simulink model "ACC_ISO_test_005_cs"  (Simulink 7.6)
settings: Solver=ode5  SolverMode=SingleTasking  StartTime=0.0  StopTime=inf  FixedStep=1/100  RelTol=1e-3
PreLoadFcn:
  | check_NUTS_defined;
  | 
  | assignin('base',['model_closed_' bdroot],false);addpath('../includes_ACC');
InitFcn:
  | PreScanExperimentInitFcn(bdroot)
StopFcn:
  | PreScanExperimentStopFcn(bdroot)
undefined symbols (not defined in the file): DiscIntNeverNeededParam, x_ini_VRML, y_ini_VRML, z_ini_VRML
libraries: simulink x25, PreScanSimulinkLibrary x12, simulink_extras x8, PreScanUsefulBlocks x5, simulink_need_slupdate x1
(part 2 of 7)

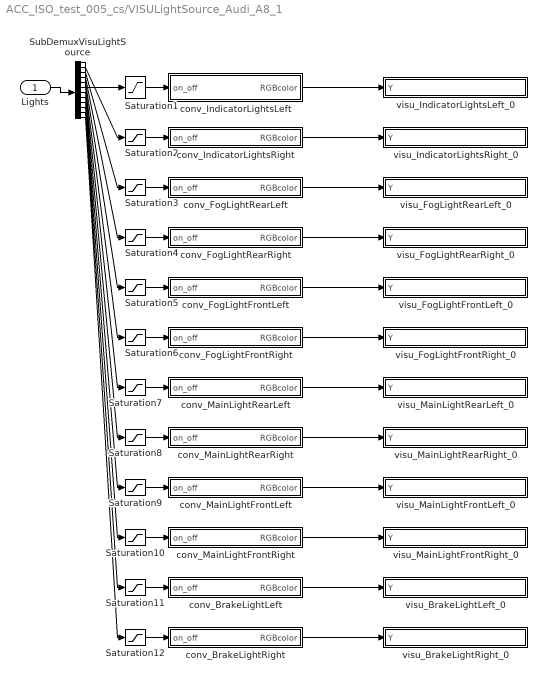
== system ACC_ISO_test_005_cs/VISULightSource_Audi_A8_1 ==
  Lights : Inport
  Saturation{1..12} (12 alike) : Saturate  UpperLimit=1  LowerLimit=0
  SubDemuxVisuLightSource : Demux  Outputs=12
  conv_BrakeLightLeft : Subsystem
  conv_BrakeLightRight : Subsystem
  conv_FogLightFrontLeft : Subsystem
  conv_FogLightFrontRight : Subsystem
  conv_FogLightRearLeft : Subsystem
  conv_FogLightRearRight : Subsystem
  conv_IndicatorLightsLeft : Subsystem
  conv_IndicatorLightsRight : Subsystem
  conv_MainLightFrontLeft : Subsystem
  conv_MainLightFrontRight : Subsystem
  conv_MainLightRearLeft : Subsystem
  conv_MainLightRearRight : Subsystem
  visu_BrakeLightLeft_0 : Subsystem  mask(ToSensorWorld){PortName=visu_BrakeLightLeft_0, PortIndex=203, PortWidth=16, TimeStep=1/100}
      mask prompts: PortName "Port Name [-]"; PortIndex "Index [-]"; PortWidth "Port Dimensions [-]"; TimeStep "Upload Period [s]"
      mask help: Sends signal(s) from Simulink to the Sensor World
      mask Help:
      | Sends signal(s) from Simulink to the Sensor World.
      | 
      | - Port Name [-]: specifies the name of the output terminal of the Simulink block.
      | - Index [-]: specifies the start position in the output vector sent to the Sensor World
      | - Port dimensions [-]: specifies the width (number of scalars) of the output port
      | - Upload period [s]: specifies the upload period (in seconds) of the port.
      mask Display: port_label('input', 1, PortName)
  visu_BrakeLightRight_0 : Subsystem  mask(ToSensorWorld){PortName=visu_BrakeLightRight_0, PortIndex=219, PortWidth=16, TimeStep=1/100}
      mask prompts: PortName "Port Name [-]"; PortIndex "Index [-]"; PortWidth "Port Dimensions [-]"; TimeStep "Upload Period [s]"
      mask help: Sends signal(s) from Simulink to the Sensor World
      mask Help:
      | Sends signal(s) from Simulink to the Sensor World.
      | 
      | - Port Name [-]: specifies the name of the output terminal of the Simulink block.
      | - Index [-]: specifies the start position in the output vector sent to the Sensor World
      | - Port dimensions [-]: specifies the width (number of scalars) of the output port
      | - Upload period [s]: specifies the upload period (in seconds) of the port.
      mask Display: port_label('input', 1, PortName)
  visu_FogLightFrontLeft_0 : Subsystem  mask(ToSensorWorld){PortName=visu_FogLightFrontLeft_0, PortIndex=107, PortWidth=16, TimeStep=1/100}
      mask prompts: PortName "Port Name [-]"; PortIndex "Index [-]"; PortWidth "Port Dimensions [-]"; TimeStep "Upload Period [s]"
      mask help: Sends signal(s) from Simulink to the Sensor World
      mask Help:
      | Sends signal(s) from Simulink to the Sensor World.
      | 
      | - Port Name [-]: specifies the name of the output terminal of the Simulink block.
      | - Index [-]: specifies the start position in the output vector sent to the Sensor World
      | - Port dimensions [-]: specifies the width (number of scalars) of the output port
      | - Upload period [s]: specifies the upload period (in seconds) of the port.
      mask Display: port_label('input', 1, PortName)
  visu_FogLightFrontRight_0 : Subsystem  mask(ToSensorWorld){PortName=visu_FogLightFrontRight_0, PortIndex=123, PortWidth=16, TimeStep=1/100}
      mask prompts: PortName "Port Name [-]"; PortIndex "Index [-]"; PortWidth "Port Dimensions [-]"; TimeStep "Upload Period [s]"
      mask help: Sends signal(s) from Simulink to the Sensor World
      mask Help:
      | Sends signal(s) from Simulink to the Sensor World.
      | 
      | - Port Name [-]: specifies the name of the output terminal of the Simulink block.
      | - Index [-]: specifies the start position in the output vector sent to the Sensor World
      | - Port dimensions [-]: specifies the width (number of scalars) of the output port
      | - Upload period [s]: specifies the upload period (in seconds) of the port.
      mask Display: port_label('input', 1, PortName)
  visu_FogLightRearLeft_0 : Subsystem  mask(ToSensorWorld){PortName=visu_FogLightRearLeft_0, PortIndex=75, PortWidth=16, TimeStep=1/100}
      mask prompts: PortName "Port Name [-]"; PortIndex "Index [-]"; PortWidth "Port Dimensions [-]"; TimeStep "Upload Period [s]"
      mask help: Sends signal(s) from Simulink to the Sensor World
      mask Help:
      | Sends signal(s) from Simulink to the Sensor World.
      | 
      | - Port Name [-]: specifies the name of the output terminal of the Simulink block.
      | - Index [-]: specifies the start position in the output vector sent to the Sensor World
      | - Port dimensions [-]: specifies the width (number of scalars) of the output port
      | - Upload period [s]: specifies the upload period (in seconds) of the port.
      mask Display: port_label('input', 1, PortName)
  visu_FogLightRearRight_0 : Subsystem  mask(ToSensorWorld){PortName=visu_FogLightRearRight_0, PortIndex=91, PortWidth=16, TimeStep=1/100}
      mask prompts: PortName "Port Name [-]"; PortIndex "Index [-]"; PortWidth "Port Dimensions [-]"; TimeStep "Upload Period [s]"
      mask help: Sends signal(s) from Simulink to the Sensor World
      mask Help:
      | Sends signal(s) from Simulink to the Sensor World.
      | 
      | - Port Name [-]: specifies the name of the output terminal of the Simulink block.
      | - Index [-]: specifies the start position in the output vector sent to the Sensor World
      | - Port dimensions [-]: specifies the width (number of scalars) of the output port
      | - Upload period [s]: specifies the upload period (in seconds) of the port.
      mask Display: port_label('input', 1, PortName)
  visu_IndicatorLightsLeft_0 : Subsystem  mask(ToSensorWorld){PortName=visu_IndicatorLightsLeft_0, PortIndex=43, PortWidth=16, TimeStep=1/100}
      mask prompts: PortName "Port Name [-]"; PortIndex "Index [-]"; PortWidth "Port Dimensions [-]"; TimeStep "Upload Period [s]"
      mask help: Sends signal(s) from Simulink to the Sensor World
      mask Help:
      | Sends signal(s) from Simulink to the Sensor World.
      | 
      | - Port Name [-]: specifies the name of the output terminal of the Simulink block.
      | - Index [-]: specifies the start position in the output vector sent to the Sensor World
      | - Port dimensions [-]: specifies the width (number of scalars) of the output port
      | - Upload period [s]: specifies the upload period (in seconds) of the port.
      mask Display: port_label('input', 1, PortName)
  visu_IndicatorLightsRight_0 : Subsystem  mask(ToSensorWorld){PortName=visu_IndicatorLightsRight_0, PortIndex=59, PortWidth=16, TimeStep=1/100}
      mask prompts: PortName "Port Name [-]"; PortIndex "Index [-]"; PortWidth "Port Dimensions [-]"; TimeStep "Upload Period [s]"
      mask help: Sends signal(s) from Simulink to the Sensor World
      mask Help:
      | Sends signal(s) from Simulink to the Sensor World.
      | 
      | - Port Name [-]: specifies the name of the output terminal of the Simulink block.
      | - Index [-]: specifies the start position in the output vector sent to the Sensor World
      | - Port dimensions [-]: specifies the width (number of scalars) of the output port
      | - Upload period [s]: specifies the upload period (in seconds) of the port.
      mask Display: port_label('input', 1, PortName)
  visu_MainLightFrontLeft_0 : Subsystem  mask(ToSensorWorld){PortName=visu_MainLightFrontLeft_0, PortIndex=171, PortWidth=16, TimeStep=1/100}
      mask prompts: PortName "Port Name [-]"; PortIndex "Index [-]"; PortWidth "Port Dimensions [-]"; TimeStep "Upload Period [s]"
      mask help: Sends signal(s) from Simulink to the Sensor World
      mask Help:
      | Sends signal(s) from Simulink to the Sensor World.
      | 
      | - Port Name [-]: specifies the name of the output terminal of the Simulink block.
      | - Index [-]: specifies the start position in the output vector sent to the Sensor World
      | - Port dimensions [-]: specifies the width (number of scalars) of the output port
      | - Upload period [s]: specifies the upload period (in seconds) of the port.
      mask Display: port_label('input', 1, PortName)
  visu_MainLightFrontRight_0 : Subsystem  mask(ToSensorWorld){PortName=visu_MainLightFrontRight_0, PortIndex=187, PortWidth=16, TimeStep=1/100}
      mask prompts: PortName "Port Name [-]"; PortIndex "Index [-]"; PortWidth "Port Dimensions [-]"; TimeStep "Upload Period [s]"
      mask help: Sends signal(s) from Simulink to the Sensor World
      mask Help:
      | Sends signal(s) from Simulink to the Sensor World.
      | 
      | - Port Name [-]: specifies the name of the output terminal of the Simulink block.
      | - Index [-]: specifies the start position in the output vector sent to the Sensor World
      | - Port dimensions [-]: specifies the width (number of scalars) of the output port
      | - Upload period [s]: specifies the upload period (in seconds) of the port.
      mask Display: port_label('input', 1, PortName)
  visu_MainLightRearLeft_0 : Subsystem  mask(ToSensorWorld){PortName=visu_MainLightRearLeft_0, PortIndex=139, PortWidth=16, TimeStep=1/100}
      mask prompts: PortName "Port Name [-]"; PortIndex "Index [-]"; PortWidth "Port Dimensions [-]"; TimeStep "Upload Period [s]"
      mask help: Sends signal(s) from Simulink to the Sensor World
      mask Help:
      | Sends signal(s) from Simulink to the Sensor World.
      | 
      | - Port Name [-]: specifies the name of the output terminal of the Simulink block.
      | - Index [-]: specifies the start position in the output vector sent to the Sensor World
      | - Port dimensions [-]: specifies the width (number of scalars) of the output port
      | - Upload period [s]: specifies the upload period (in seconds) of the port.
      mask Display: port_label('input', 1, PortName)
  visu_MainLightRearRight_0 : Subsystem  mask(ToSensorWorld){PortName=visu_MainLightRearRight_0, PortIndex=155, PortWidth=16, TimeStep=1/100}
      mask prompts: PortName "Port Name [-]"; PortIndex "Index [-]"; PortWidth "Port Dimensions [-]"; TimeStep "Upload Period [s]"
      mask help: Sends signal(s) from Simulink to the Sensor World
      mask Help:
      | Sends signal(s) from Simulink to the Sensor World.
      | 
      | - Port Name [-]: specifies the name of the output terminal of the Simulink block.
      | - Index [-]: specifies the start position in the output vector sent to the Sensor World
      | - Port dimensions [-]: specifies the width (number of scalars) of the output port
      | - Upload period [s]: specifies the upload period (in seconds) of the port.
      mask Display: port_label('input', 1, PortName)
  wires:
  Lights/1 -> SubDemuxVisuLightSource/1
  SubDemuxVisuLightSource/1 -> Saturation1/1
  Saturation1/1 -> conv_IndicatorLightsLeft/1(on_off)
  conv_IndicatorLightsLeft/1(RGBcolor) -> visu_IndicatorLightsLeft_0/1(Y)
  SubDemuxVisuLightSource/2 -> Saturation2/1
  Saturation2/1 -> conv_IndicatorLightsRight/1(on_off)
  conv_IndicatorLightsRight/1(RGBcolor) -> visu_IndicatorLightsRight_0/1(Y)
  SubDemuxVisuLightSource/3 -> Saturation3/1
  Saturation3/1 -> conv_FogLightRearLeft/1(on_off)
  conv_FogLightRearLeft/1(RGBcolor) -> visu_FogLightRearLeft_0/1(Y)
  SubDemuxVisuLightSource/4 -> Saturation4/1
  Saturation4/1 -> conv_FogLightRearRight/1(on_off)
  conv_FogLightRearRight/1(RGBcolor) -> visu_FogLightRearRight_0/1(Y)
  SubDemuxVisuLightSource/5 -> Saturation5/1
  Saturation5/1 -> conv_FogLightFrontLeft/1(on_off)
  conv_FogLightFrontLeft/1(RGBcolor) -> visu_FogLightFrontLeft_0/1(Y)
  SubDemuxVisuLightSource/6 -> Saturation6/1
  Saturation6/1 -> conv_FogLightFrontRight/1(on_off)
  conv_FogLightFrontRight/1(RGBcolor) -> visu_FogLightFrontRight_0/1(Y)
  SubDemuxVisuLightSource/7 -> Saturation7/1
  Saturation7/1 -> conv_MainLightRearLeft/1(on_off)
  conv_MainLightRearLeft/1(RGBcolor) -> visu_MainLightRearLeft_0/1(Y)
  SubDemuxVisuLightSource/8 -> Saturation8/1
  Saturation8/1 -> conv_MainLightRearRight/1(on_off)
  conv_MainLightRearRight/1(RGBcolor) -> visu_MainLightRearRight_0/1(Y)
  SubDemuxVisuLightSource/9 -> Saturation9/1
  Saturation9/1 -> conv_MainLightFrontLeft/1(on_off)
  conv_MainLightFrontLeft/1(RGBcolor) -> visu_MainLightFrontLeft_0/1(Y)
  SubDemuxVisuLightSource/10 -> Saturation10/1
  Saturation10/1 -> conv_MainLightFrontRight/1(on_off)
  conv_MainLightFrontRight/1(RGBcolor) -> visu_MainLightFrontRight_0/1(Y)
  SubDemuxVisuLightSource/11 -> Saturation11/1
  Saturation11/1 -> conv_BrakeLightLeft/1(on_off)
  conv_BrakeLightLeft/1(RGBcolor) -> visu_BrakeLightLeft_0/1(Y)
  SubDemuxVisuLightSource/12 -> Saturation12/1
  Saturation12/1 -> conv_BrakeLightRight/1(on_off)
  conv_BrakeLightRight/1(RGBcolor) -> visu_BrakeLightRight_0/1(Y)

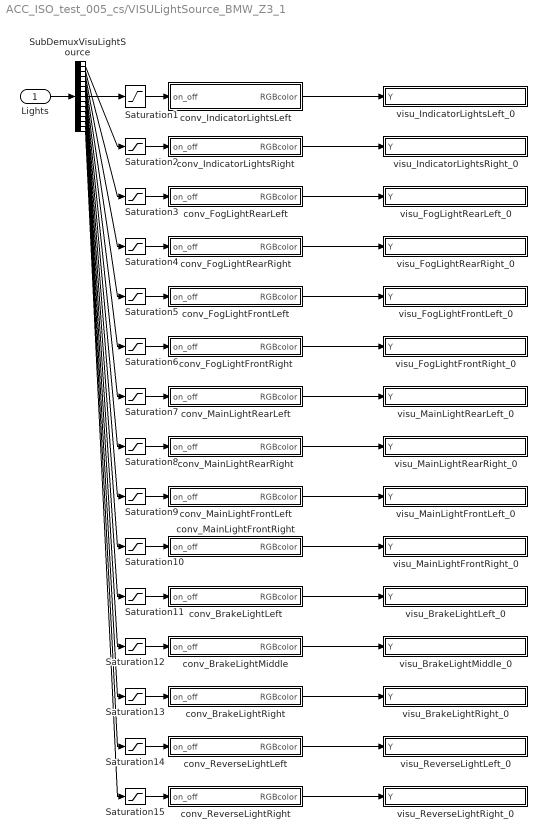
== system ACC_ISO_test_005_cs/VISULightSource_BMW_Z3_1 ==
  Lights : Inport
  Saturation{1..15} (15 alike) : Saturate  UpperLimit=1  LowerLimit=0
  SubDemuxVisuLightSource : Demux  Outputs=15
  conv_BrakeLightLeft : Subsystem
  conv_BrakeLightMiddle : Subsystem
  conv_BrakeLightRight : Subsystem
  conv_FogLightFrontLeft : Subsystem
  conv_FogLightFrontRight : Subsystem
  conv_FogLightRearLeft : Subsystem
  conv_FogLightRearRight : Subsystem
  conv_IndicatorLightsLeft : Subsystem
  conv_IndicatorLightsRight : Subsystem
  conv_MainLightFrontLeft : Subsystem
  conv_MainLightFrontRight : Subsystem
  conv_MainLightRearLeft : Subsystem
  conv_MainLightRearRight : Subsystem
  conv_ReverseLightLeft : Subsystem
  conv_ReverseLightRight : Subsystem
  visu_BrakeLightLeft_0 : Subsystem  mask(ToSensorWorld){PortName=visu_BrakeLightLeft_0, PortIndex=461, PortWidth=16, TimeStep=1/100}
      mask prompts: PortName "Port Name [-]"; PortIndex "Index [-]"; PortWidth "Port Dimensions [-]"; TimeStep "Upload Period [s]"
      mask help: Sends signal(s) from Simulink to the Sensor World
      mask Help:
      | Sends signal(s) from Simulink to the Sensor World.
      | 
      | - Port Name [-]: specifies the name of the output terminal of the Simulink block.
      | - Index [-]: specifies the start position in the output vector sent to the Sensor World
      | - Port dimensions [-]: specifies the width (number of scalars) of the output port
      | - Upload period [s]: specifies the upload period (in seconds) of the port.
      mask Display: port_label('input', 1, PortName)
  visu_BrakeLightMiddle_0 : Subsystem  mask(ToSensorWorld){PortName=visu_BrakeLightMiddle_0, PortIndex=477, PortWidth=16, TimeStep=1/100}
      mask prompts: PortName "Port Name [-]"; PortIndex "Index [-]"; PortWidth "Port Dimensions [-]"; TimeStep "Upload Period [s]"
      mask help: Sends signal(s) from Simulink to the Sensor World
      mask Help:
      | Sends signal(s) from Simulink to the Sensor World.
      | 
      | - Port Name [-]: specifies the name of the output terminal of the Simulink block.
      | - Index [-]: specifies the start position in the output vector sent to the Sensor World
      | - Port dimensions [-]: specifies the width (number of scalars) of the output port
      | - Upload period [s]: specifies the upload period (in seconds) of the port.
      mask Display: port_label('input', 1, PortName)
  visu_BrakeLightRight_0 : Subsystem  mask(ToSensorWorld){PortName=visu_BrakeLightRight_0, PortIndex=493, PortWidth=16, TimeStep=1/100}
      mask prompts: PortName "Port Name [-]"; PortIndex "Index [-]"; PortWidth "Port Dimensions [-]"; TimeStep "Upload Period [s]"
      mask help: Sends signal(s) from Simulink to the Sensor World
      mask Help:
      | Sends signal(s) from Simulink to the Sensor World.
      | 
      | - Port Name [-]: specifies the name of the output terminal of the Simulink block.
      | - Index [-]: specifies the start position in the output vector sent to the Sensor World
      | - Port dimensions [-]: specifies the width (number of scalars) of the output port
      | - Upload period [s]: specifies the upload period (in seconds) of the port.
      mask Display: port_label('input', 1, PortName)
  visu_FogLightFrontLeft_0 : Subsystem  mask(ToSensorWorld){PortName=visu_FogLightFrontLeft_0, PortIndex=365, PortWidth=16, TimeStep=1/100}
      mask prompts: PortName "Port Name [-]"; PortIndex "Index [-]"; PortWidth "Port Dimensions [-]"; TimeStep "Upload Period [s]"
      mask help: Sends signal(s) from Simulink to the Sensor World
      mask Help:
      | Sends signal(s) from Simulink to the Sensor World.
      | 
      | - Port Name [-]: specifies the name of the output terminal of the Simulink block.
      | - Index [-]: specifies the start position in the output vector sent to the Sensor World
      | - Port dimensions [-]: specifies the width (number of scalars) of the output port
      | - Upload period [s]: specifies the upload period (in seconds) of the port.
      mask Display: port_label('input', 1, PortName)
  visu_FogLightFrontRight_0 : Subsystem  mask(ToSensorWorld){PortName=visu_FogLightFrontRight_0, PortIndex=381, PortWidth=16, TimeStep=1/100}
      mask prompts: PortName "Port Name [-]"; PortIndex "Index [-]"; PortWidth "Port Dimensions [-]"; TimeStep "Upload Period [s]"
      mask help: Sends signal(s) from Simulink to the Sensor World
      mask Help:
      | Sends signal(s) from Simulink to the Sensor World.
      | 
      | - Port Name [-]: specifies the name of the output terminal of the Simulink block.
      | - Index [-]: specifies the start position in the output vector sent to the Sensor World
      | - Port dimensions [-]: specifies the width (number of scalars) of the output port
      | - Upload period [s]: specifies the upload period (in seconds) of the port.
      mask Display: port_label('input', 1, PortName)
  visu_FogLightRearLeft_0 : Subsystem  mask(ToSensorWorld){PortName=visu_FogLightRearLeft_0, PortIndex=333, PortWidth=16, TimeStep=1/100}
      mask prompts: PortName "Port Name [-]"; PortIndex "Index [-]"; PortWidth "Port Dimensions [-]"; TimeStep "Upload Period [s]"
      mask help: Sends signal(s) from Simulink to the Sensor World
      mask Help:
      | Sends signal(s) from Simulink to the Sensor World.
      | 
      | - Port Name [-]: specifies the name of the output terminal of the Simulink block.
      | - Index [-]: specifies the start position in the output vector sent to the Sensor World
      | - Port dimensions [-]: specifies the width (number of scalars) of the output port
      | - Upload period [s]: specifies the upload period (in seconds) of the port.
      mask Display: port_label('input', 1, PortName)
  visu_FogLightRearRight_0 : Subsystem  mask(ToSensorWorld){PortName=visu_FogLightRearRight_0, PortIndex=349, PortWidth=16, TimeStep=1/100}
      mask prompts: PortName "Port Name [-]"; PortIndex "Index [-]"; PortWidth "Port Dimensions [-]"; TimeStep "Upload Period [s]"
      mask help: Sends signal(s) from Simulink to the Sensor World
      mask Help:
      | Sends signal(s) from Simulink to the Sensor World.
      | 
      | - Port Name [-]: specifies the name of the output terminal of the Simulink block.
      | - Index [-]: specifies the start position in the output vector sent to the Sensor World
      | - Port dimensions [-]: specifies the width (number of scalars) of the output port
      | - Upload period [s]: specifies the upload period (in seconds) of the port.
      mask Display: port_label('input', 1, PortName)
  visu_IndicatorLightsLeft_0 : Subsystem  mask(ToSensorWorld){PortName=visu_IndicatorLightsLeft_0, PortIndex=301, PortWidth=16, TimeStep=1/100}
      mask prompts: PortName "Port Name [-]"; PortIndex "Index [-]"; PortWidth "Port Dimensions [-]"; TimeStep "Upload Period [s]"
      mask help: Sends signal(s) from Simulink to the Sensor World
      mask Help:
      | Sends signal(s) from Simulink to the Sensor World.
      | 
      | - Port Name [-]: specifies the name of the output terminal of the Simulink block.
      | - Index [-]: specifies the start position in the output vector sent to the Sensor World
      | - Port dimensions [-]: specifies the width (number of scalars) of the output port
      | - Upload period [s]: specifies the upload period (in seconds) of the port.
      mask Display: port_label('input', 1, PortName)
  visu_IndicatorLightsRight_0 : Subsystem  mask(ToSensorWorld){PortName=visu_IndicatorLightsRight_0, PortIndex=317, PortWidth=16, TimeStep=1/100}
      mask prompts: PortName "Port Name [-]"; PortIndex "Index [-]"; PortWidth "Port Dimensions [-]"; TimeStep "Upload Period [s]"
      mask help: Sends signal(s) from Simulink to the Sensor World
      mask Help:
      | Sends signal(s) from Simulink to the Sensor World.
      | 
      | - Port Name [-]: specifies the name of the output terminal of the Simulink block.
      | - Index [-]: specifies the start position in the output vector sent to the Sensor World
      | - Port dimensions [-]: specifies the width (number of scalars) of the output port
      | - Upload period [s]: specifies the upload period (in seconds) of the port.
      mask Display: port_label('input', 1, PortName)
  visu_MainLightFrontLeft_0 : Subsystem  mask(ToSensorWorld){PortName=visu_MainLightFrontLeft_0, PortIndex=429, PortWidth=16, TimeStep=1/100}
      mask prompts: PortName "Port Name [-]"; PortIndex "Index [-]"; PortWidth "Port Dimensions [-]"; TimeStep "Upload Period [s]"
      mask help: Sends signal(s) from Simulink to the Sensor World
      mask Help:
      | Sends signal(s) from Simulink to the Sensor World.
      | 
      | - Port Name [-]: specifies the name of the output terminal of the Simulink block.
      | - Index [-]: specifies the start position in the output vector sent to the Sensor World
      | - Port dimensions [-]: specifies the width (number of scalars) of the output port
      | - Upload period [s]: specifies the upload period (in seconds) of the port.
      mask Display: port_label('input', 1, PortName)
  visu_MainLightFrontRight_0 : Subsystem  mask(ToSensorWorld){PortName=visu_MainLightFrontRight_0, PortIndex=445, PortWidth=16, TimeStep=1/100}
      mask prompts: PortName "Port Name [-]"; PortIndex "Index [-]"; PortWidth "Port Dimensions [-]"; TimeStep "Upload Period [s]"
      mask help: Sends signal(s) from Simulink to the Sensor World
      mask Help:
      | Sends signal(s) from Simulink to the Sensor World.
      | 
      | - Port Name [-]: specifies the name of the output terminal of the Simulink block.
      | - Index [-]: specifies the start position in the output vector sent to the Sensor World
      | - Port dimensions [-]: specifies the width (number of scalars) of the output port
      | - Upload period [s]: specifies the upload period (in seconds) of the port.
      mask Display: port_label('input', 1, PortName)
  visu_MainLightRearLeft_0 : Subsystem  mask(ToSensorWorld){PortName=visu_MainLightRearLeft_0, PortIndex=397, PortWidth=16, TimeStep=1/100}
      mask prompts: PortName "Port Name [-]"; PortIndex "Index [-]"; PortWidth "Port Dimensions [-]"; TimeStep "Upload Period [s]"
      mask help: Sends signal(s) from Simulink to the Sensor World
      mask Help:
      | Sends signal(s) from Simulink to the Sensor World.
      | 
      | - Port Name [-]: specifies the name of the output terminal of the Simulink block.
      | - Index [-]: specifies the start position in the output vector sent to the Sensor World
      | - Port dimensions [-]: specifies the width (number of scalars) of the output port
      | - Upload period [s]: specifies the upload period (in seconds) of the port.
      mask Display: port_label('input', 1, PortName)
  visu_MainLightRearRight_0 : Subsystem  mask(ToSensorWorld){PortName=visu_MainLightRearRight_0, PortIndex=413, PortWidth=16, TimeStep=1/100}
      mask prompts: PortName "Port Name [-]"; PortIndex "Index [-]"; PortWidth "Port Dimensions [-]"; TimeStep "Upload Period [s]"
      mask help: Sends signal(s) from Simulink to the Sensor World
      mask Help:
      | Sends signal(s) from Simulink to the Sensor World.
      | 
      | - Port Name [-]: specifies the name of the output terminal of the Simulink block.
      | - Index [-]: specifies the start position in the output vector sent to the Sensor World
      | - Port dimensions [-]: specifies the width (number of scalars) of the output port
      | - Upload period [s]: specifies the upload period (in seconds) of the port.
      mask Display: port_label('input', 1, PortName)
  visu_ReverseLightLeft_0 : Subsystem  mask(ToSensorWorld){PortName=visu_ReverseLightLeft_0, PortIndex=509, PortWidth=16, TimeStep=1/100}
      mask prompts: PortName "Port Name [-]"; PortIndex "Index [-]"; PortWidth "Port Dimensions [-]"; TimeStep "Upload Period [s]"
      mask help: Sends signal(s) from Simulink to the Sensor World
      mask Help:
      | Sends signal(s) from Simulink to the Sensor World.
      | 
      | - Port Name [-]: specifies the name of the output terminal of the Simulink block.
      | - Index [-]: specifies the start position in the output vector sent to the Sensor World
      | - Port dimensions [-]: specifies the width (number of scalars) of the output port
      | - Upload period [s]: specifies the upload period (in seconds) of the port.
      mask Display: port_label('input', 1, PortName)
  visu_ReverseLightRight_0 : Subsystem  mask(ToSensorWorld){PortName=visu_ReverseLightRight_0, PortIndex=525, PortWidth=16, TimeStep=1/100}
      mask prompts: PortName "Port Name [-]"; PortIndex "Index [-]"; PortWidth "Port Dimensions [-]"; TimeStep "Upload Period [s]"
      mask help: Sends signal(s) from Simulink to the Sensor World
      mask Help:
      | Sends signal(s) from Simulink to the Sensor World.
      | 
      | - Port Name [-]: specifies the name of the output terminal of the Simulink block.
      | - Index [-]: specifies the start position in the output vector sent to the Sensor World
      | - Port dimensions [-]: specifies the width (number of scalars) of the output port
      | - Upload period [s]: specifies the upload period (in seconds) of the port.
      mask Display: port_label('input', 1, PortName)
  wires:
  Lights/1 -> SubDemuxVisuLightSource/1
  SubDemuxVisuLightSource/1 -> Saturation1/1
  Saturation1/1 -> conv_IndicatorLightsLeft/1(on_off)
  conv_IndicatorLightsLeft/1(RGBcolor) -> visu_IndicatorLightsLeft_0/1(Y)
  SubDemuxVisuLightSource/2 -> Saturation2/1
  Saturation2/1 -> conv_IndicatorLightsRight/1(on_off)
  conv_IndicatorLightsRight/1(RGBcolor) -> visu_IndicatorLightsRight_0/1(Y)
  SubDemuxVisuLightSource/3 -> Saturation3/1
  Saturation3/1 -> conv_FogLightRearLeft/1(on_off)
  conv_FogLightRearLeft/1(RGBcolor) -> visu_FogLightRearLeft_0/1(Y)
  SubDemuxVisuLightSource/4 -> Saturation4/1
  Saturation4/1 -> conv_FogLightRearRight/1(on_off)
  conv_FogLightRearRight/1(RGBcolor) -> visu_FogLightRearRight_0/1(Y)
  SubDemuxVisuLightSource/5 -> Saturation5/1
  Saturation5/1 -> conv_FogLightFrontLeft/1(on_off)
  conv_FogLightFrontLeft/1(RGBcolor) -> visu_FogLightFrontLeft_0/1(Y)
  SubDemuxVisuLightSource/6 -> Saturation6/1
  Saturation6/1 -> conv_FogLightFrontRight/1(on_off)
  conv_FogLightFrontRight/1(RGBcolor) -> visu_FogLightFrontRight_0/1(Y)
  SubDemuxVisuLightSource/7 -> Saturation7/1
  Saturation7/1 -> conv_MainLightRearLeft/1(on_off)
  conv_MainLightRearLeft/1(RGBcolor) -> visu_MainLightRearLeft_0/1(Y)
  SubDemuxVisuLightSource/8 -> Saturation8/1
  Saturation8/1 -> conv_MainLightRearRight/1(on_off)
  conv_MainLightRearRight/1(RGBcolor) -> visu_MainLightRearRight_0/1(Y)
  SubDemuxVisuLightSource/9 -> Saturation9/1
  Saturation9/1 -> conv_MainLightFrontLeft/1(on_off)
  conv_MainLightFrontLeft/1(RGBcolor) -> visu_MainLightFrontLeft_0/1(Y)
  SubDemuxVisuLightSource/10 -> Saturation10/1
  Saturation10/1 -> conv_MainLightFrontRight/1(on_off)
  conv_MainLightFrontRight/1(RGBcolor) -> visu_MainLightFrontRight_0/1(Y)
  SubDemuxVisuLightSource/11 -> Saturation11/1
  Saturation11/1 -> conv_BrakeLightLeft/1(on_off)
  conv_BrakeLightLeft/1(RGBcolor) -> visu_BrakeLightLeft_0/1(Y)
  SubDemuxVisuLightSource/12 -> Saturation12/1
  Saturation12/1 -> conv_BrakeLightMiddle/1(on_off)
  conv_BrakeLightMiddle/1(RGBcolor) -> visu_BrakeLightMiddle_0/1(Y)
  SubDemuxVisuLightSource/13 -> Saturation13/1
  Saturation13/1 -> conv_BrakeLightRight/1(on_off)
  conv_BrakeLightRight/1(RGBcolor) -> visu_BrakeLightRight_0/1(Y)
  SubDemuxVisuLightSource/14 -> Saturation14/1
  Saturation14/1 -> conv_ReverseLightLeft/1(on_off)
  conv_ReverseLightLeft/1(RGBcolor) -> visu_ReverseLightLeft_0/1(Y)
  SubDemuxVisuLightSource/15 -> Saturation15/1
  Saturation15/1 -> conv_ReverseLightRight/1(on_off)
  conv_ReverseLightRight/1(RGBcolor) -> visu_ReverseLightRight_0/1(Y)

== system ACC_ISO_test_005_cs/VISUSteer_Audi_A8_1 ==
  Steer : Inport
  Demux3 : Demux  Outputs=[1 1]
  Saturation : Saturate  UpperLimit=30  LowerLimit=-5
  Saturation1 : Saturate  UpperLimit=720  LowerLimit=-720
  conv_SteeringColumn : Subsystem
  conv_SteeringWheel : Subsystem
  visu_SteeringColumn : Subsystem  mask(ToSensorWorld){PortName=visu_SteeringColumn_0, PortIndex=239, PortWidth=4, TimeStep=1/100}
      mask prompts: PortName "Port Name [-]"; PortIndex "Index [-]"; PortWidth "Port Dimensions [-]"; TimeStep "Upload Period [s]"
      mask help: Sends signal(s) from Simulink to the Sensor World
      mask Help:
      | Sends signal(s) from Simulink to the Sensor World.
      | 
      | - Port Name [-]: specifies the name of the output terminal of the Simulink block.
      | - Index [-]: specifies the start position in the output vector sent to the Sensor World
      | - Port dimensions [-]: specifies the width (number of scalars) of the output port
      | - Upload period [s]: specifies the upload period (in seconds) of the port.
      mask Display: port_label('input', 1, PortName)
  visu_SteeringWheel : Subsystem  mask(ToSensorWorld){PortName=visu_SteeringWheel_0, PortIndex=235, PortWidth=4, TimeStep=1/100}
      mask prompts: PortName "Port Name [-]"; PortIndex "Index [-]"; PortWidth "Port Dimensions [-]"; TimeStep "Upload Period [s]"
      mask help: Sends signal(s) from Simulink to the Sensor World
      mask Help:
      | Sends signal(s) from Simulink to the Sensor World.
      | 
      | - Port Name [-]: specifies the name of the output terminal of the Simulink block.
      | - Index [-]: specifies the start position in the output vector sent to the Sensor World
      | - Port dimensions [-]: specifies the width (number of scalars) of the output port
      | - Upload period [s]: specifies the upload period (in seconds) of the port.
      mask Display: port_label('input', 1, PortName)
  wires:
  conv_SteeringColumn/1(QuaternionVisu [rad]) -> visu_SteeringColumn/1(Y)
  conv_SteeringWheel/1(QuaternionVisu [rad]) -> visu_SteeringWheel/1(Y)
  Demux3/2 -> Saturation/1
  Demux3/1 -> Saturation1/1
  Saturation1/1 -> conv_SteeringWheel/1(angle [deg])
  Saturation/1 -> conv_SteeringColumn/1(angle [deg])
  Steer/1 -> Demux3/1

== system ACC_ISO_test_005_cs/VISUSteer_BMW_Z3_1 ==
  Steer : Inport
  Demux3 : Demux  Outputs=[1 1]
  Saturation : Saturate  UpperLimit=30  LowerLimit=-5
  Saturation1 : Saturate  UpperLimit=720  LowerLimit=-720
  conv_SteeringColumn : Subsystem
  conv_SteeringWheel : Subsystem
  visu_SteeringColumn : Subsystem  mask(ToSensorWorld){PortName=visu_SteeringColumn_0, PortIndex=545, PortWidth=4, TimeStep=1/100}
      mask prompts: PortName "Port Name [-]"; PortIndex "Index [-]"; PortWidth "Port Dimensions [-]"; TimeStep "Upload Period [s]"
      mask help: Sends signal(s) from Simulink to the Sensor World
      mask Help:
      | Sends signal(s) from Simulink to the Sensor World.
      | 
      | - Port Name [-]: specifies the name of the output terminal of the Simulink block.
      | - Index [-]: specifies the start position in the output vector sent to the Sensor World
      | - Port dimensions [-]: specifies the width (number of scalars) of the output port
      | - Upload period [s]: specifies the upload period (in seconds) of the port.
      mask Display: port_label('input', 1, PortName)
  visu_SteeringWheel : Subsystem  mask(ToSensorWorld){PortName=visu_SteeringWheel_0, PortIndex=541, PortWidth=4, TimeStep=1/100}
      mask prompts: PortName "Port Name [-]"; PortIndex "Index [-]"; PortWidth "Port Dimensions [-]"; TimeStep "Upload Period [s]"
      mask help: Sends signal(s) from Simulink to the Sensor World
      mask Help:
      | Sends signal(s) from Simulink to the Sensor World.
      | 
      | - Port Name [-]: specifies the name of the output terminal of the Simulink block.
      | - Index [-]: specifies the start position in the output vector sent to the Sensor World
      | - Port dimensions [-]: specifies the width (number of scalars) of the output port
      | - Upload period [s]: specifies the upload period (in seconds) of the port.
      mask Display: port_label('input', 1, PortName)
  wires:
  conv_SteeringColumn/1(QuaternionVisu [rad]) -> visu_SteeringColumn/1(Y)
  conv_SteeringWheel/1(QuaternionVisu [rad]) -> visu_SteeringWheel/1(Y)
  Demux3/2 -> Saturation/1
  Demux3/1 -> Saturation1/1
  Saturation1/1 -> conv_SteeringWheel/1(angle [deg])
  Saturation/1 -> conv_SteeringColumn/1(angle [deg])
  Steer/1 -> Demux3/1

== system ACC_ISO_test_005_cs/VISUWheels_Audi_A8_1 ==
  Wheels : Inport
  Demux : Demux  Outputs=[3 3 3 3 3 3 3 3]
  Saturation{,2,4,6} (4 alike) : Saturate  UpperLimit=[0.2 0.2 0.5]  LowerLimit=[-0.2 -0.2 -0.5]
  Saturation{1,3,5,8} (4 alike) : Saturate  UpperLimit=[30 inf 30]  LowerLimit=[-30 -inf -30]
  conv_RotWheelFL : Subsystem
  conv_RotWheelFR : Subsystem
  conv_RotWheelRL : Subsystem
  conv_RotWheelRR : Subsystem
  conv_TransWheelFL : Subsystem  mask(Translation node configuration){tp=Front-Left Wheel, gains=off, Gain_xISO=1, Gain_yISO=1, Gain_zISO=1}
      mask prompts: tp "Type"; gains "Edit scaling factors?"; Gain_xISO "Scaling factor in x-direction (ISO-convention)"; Gain_yISO "Scaling factor in y-direction (ISO-convention)"; Gain_zISO "Scaling factor in z-direction (ISO-convention)"
      mask init:
      | Visu_ini_param('Audi_A8',tp);
      mask StyleString: popup(Front-Left Wheel|Front-Right Wheel|Rear-Left Wheel|Rear-Right Wheel|Left Seat|Right Seat),checkbox,edit,edit,edit
      mask CallbackString:
      | |if strcmp(get_param(gcb, 'gains'),'on')
      |     set_param(gcb,'MaskVisibilities',{'on','on','on','on','on'})
      | else
      |     set_param(gcb,'MaskVisibilities',{'on','on','off','off','off'})
      | end|||
  conv_TransWheelFR : Subsystem  mask(Translation node configuration){tp=Front-Right Wheel, gains=off, Gain_xISO=1, Gain_yISO=1, Gain_zISO=1}
      mask prompts: tp "Type"; gains "Edit scaling factors?"; Gain_xISO "Scaling factor in x-direction (ISO-convention)"; Gain_yISO "Scaling factor in y-direction (ISO-convention)"; Gain_zISO "Scaling factor in z-direction (ISO-convention)"
      mask init:
      | Visu_ini_param('Audi_A8',tp);
      mask StyleString: popup(Front-Left Wheel|Front-Right Wheel|Rear-Left Wheel|Rear-Right Wheel|Left Seat|Right Seat),checkbox,edit,edit,edit
      mask CallbackString:
      | |if strcmp(get_param(gcb, 'gains'),'on')
      |     set_param(gcb,'MaskVisibilities',{'on','on','on','on','on'})
      | else
      |     set_param(gcb,'MaskVisibilities',{'on','on','off','off','off'})
      | end|||
  conv_TransWheelRL : Subsystem  mask(Translation node configuration){tp=Rear-Left Wheel, gains=off, Gain_xISO=1, Gain_yISO=1, Gain_zISO=1}
      mask prompts: tp "Type"; gains "Edit scaling factors?"; Gain_xISO "Scaling factor in x-direction (ISO-convention)"; Gain_yISO "Scaling factor in y-direction (ISO-convention)"; Gain_zISO "Scaling factor in z-direction (ISO-convention)"
      mask init:
      | Visu_ini_param('Audi_A8',tp);
      mask StyleString: popup(Front-Left Wheel|Front-Right Wheel|Rear-Left Wheel|Rear-Right Wheel|Left Seat|Right Seat),checkbox,edit,edit,edit
      mask CallbackString:
      | |if strcmp(get_param(gcb, 'gains'),'on')
      |     set_param(gcb,'MaskVisibilities',{'on','on','on','on','on'})
      | else
      |     set_param(gcb,'MaskVisibilities',{'on','on','off','off','off'})
      | end|||
  conv_TransWheelRR : Subsystem  mask(Translation node configuration){tp=Rear-Right Wheel, gains=off, Gain_xISO=1, Gain_yISO=1, Gain_zISO=1}
      mask prompts: tp "Type"; gains "Edit scaling factors?"; Gain_xISO "Scaling factor in x-direction (ISO-convention)"; Gain_yISO "Scaling factor in y-direction (ISO-convention)"; Gain_zISO "Scaling factor in z-direction (ISO-convention)"
      mask init:
      | Visu_ini_param('Audi_A8',tp);
      mask StyleString: popup(Front-Left Wheel|Front-Right Wheel|Rear-Left Wheel|Rear-Right Wheel|Left Seat|Right Seat),checkbox,edit,edit,edit
      mask CallbackString:
      | |if strcmp(get_param(gcb, 'gains'),'on')
      |     set_param(gcb,'MaskVisibilities',{'on','on','on','on','on'})
      | else
      |     set_param(gcb,'MaskVisibilities',{'on','on','off','off','off'})
      | end|||
  visu_RotWheelFL : Subsystem  mask(ToSensorWorld){PortName=visu_RotWheelFL_0, PortIndex=18, PortWidth=4, TimeStep=1/100}
      mask prompts: PortName "Port Name [-]"; PortIndex "Index [-]"; PortWidth "Port Dimensions [-]"; TimeStep "Upload Period [s]"
      mask help: Sends signal(s) from Simulink to the Sensor World
      mask Help:
      | Sends signal(s) from Simulink to the Sensor World.
      | 
      | - Port Name [-]: specifies the name of the output terminal of the Simulink block.
      | - Index [-]: specifies the start position in the output vector sent to the Sensor World
      | - Port dimensions [-]: specifies the width (number of scalars) of the output port
      | - Upload period [s]: specifies the upload period (in seconds) of the port.
      mask Display: port_label('input', 1, PortName)
  visu_RotWheelFR : Subsystem  mask(ToSensorWorld){PortName=visu_RotWheelFR_0, PortIndex=25, PortWidth=4, TimeStep=1/100}
      mask prompts: PortName "Port Name [-]"; PortIndex "Index [-]"; PortWidth "Port Dimensions [-]"; TimeStep "Upload Period [s]"
      mask help: Sends signal(s) from Simulink to the Sensor World
      mask Help:
      | Sends signal(s) from Simulink to the Sensor World.
      | 
      | - Port Name [-]: specifies the name of the output terminal of the Simulink block.
      | - Index [-]: specifies the start position in the output vector sent to the Sensor World
      | - Port dimensions [-]: specifies the width (number of scalars) of the output port
      | - Upload period [s]: specifies the upload period (in seconds) of the port.
      mask Display: port_label('input', 1, PortName)
  visu_RotWheelRL : Subsystem  mask(ToSensorWorld){PortName=visu_RotWheelRL_0, PortIndex=32, PortWidth=4, TimeStep=1/100}
      mask prompts: PortName "Port Name [-]"; PortIndex "Index [-]"; PortWidth "Port Dimensions [-]"; TimeStep "Upload Period [s]"
      mask help: Sends signal(s) from Simulink to the Sensor World
      mask Help:
      | Sends signal(s) from Simulink to the Sensor World.
      | 
      | - Port Name [-]: specifies the name of the output terminal of the Simulink block.
      | - Index [-]: specifies the start position in the output vector sent to the Sensor World
      | - Port dimensions [-]: specifies the width (number of scalars) of the output port
      | - Upload period [s]: specifies the upload period (in seconds) of the port.
      mask Display: port_label('input', 1, PortName)
  visu_RotWheelRR : Subsystem  mask(ToSensorWorld){PortName=visu_RotWheelRR_0, PortIndex=39, PortWidth=4, TimeStep=1/100}
      mask prompts: PortName "Port Name [-]"; PortIndex "Index [-]"; PortWidth "Port Dimensions [-]"; TimeStep "Upload Period [s]"
      mask help: Sends signal(s) from Simulink to the Sensor World
      mask Help:
      | Sends signal(s) from Simulink to the Sensor World.
      | 
      | - Port Name [-]: specifies the name of the output terminal of the Simulink block.
      | - Index [-]: specifies the start position in the output vector sent to the Sensor World
      | - Port dimensions [-]: specifies the width (number of scalars) of the output port
      | - Upload period [s]: specifies the upload period (in seconds) of the port.
      mask Display: port_label('input', 1, PortName)
  visu_TransWheelFL : Subsystem  mask(ToSensorWorld){PortName=visu_TransWheelFL_0, PortIndex=15, PortWidth=3, TimeStep=1/100}
      mask prompts: PortName "Port Name [-]"; PortIndex "Index [-]"; PortWidth "Port Dimensions [-]"; TimeStep "Upload Period [s]"
      mask help: Sends signal(s) from Simulink to the Sensor World
      mask Help:
      | Sends signal(s) from Simulink to the Sensor World.
      | 
      | - Port Name [-]: specifies the name of the output terminal of the Simulink block.
      | - Index [-]: specifies the start position in the output vector sent to the Sensor World
      | - Port dimensions [-]: specifies the width (number of scalars) of the output port
      | - Upload period [s]: specifies the upload period (in seconds) of the port.
      mask Display: port_label('input', 1, PortName)
  visu_TransWheelFR : Subsystem  mask(ToSensorWorld){PortName=visu_TransWheelFR_0, PortIndex=22, PortWidth=3, TimeStep=1/100}
      mask prompts: PortName "Port Name [-]"; PortIndex "Index [-]"; PortWidth "Port Dimensions [-]"; TimeStep "Upload Period [s]"
      mask help: Sends signal(s) from Simulink to the Sensor World
      mask Help:
      | Sends signal(s) from Simulink to the Sensor World.
      | 
      | - Port Name [-]: specifies the name of the output terminal of the Simulink block.
      | - Index [-]: specifies the start position in the output vector sent to the Sensor World
      | - Port dimensions [-]: specifies the width (number of scalars) of the output port
      | - Upload period [s]: specifies the upload period (in seconds) of the port.
      mask Display: port_label('input', 1, PortName)
  visu_TransWheelRL : Subsystem  mask(ToSensorWorld){PortName=visu_TransWheelRL_0, PortIndex=29, PortWidth=3, TimeStep=1/100}
      mask prompts: PortName "Port Name [-]"; PortIndex "Index [-]"; PortWidth "Port Dimensions [-]"; TimeStep "Upload Period [s]"
      mask help: Sends signal(s) from Simulink to the Sensor World
      mask Help:
      | Sends signal(s) from Simulink to the Sensor World.
      | 
      | - Port Name [-]: specifies the name of the output terminal of the Simulink block.
      | - Index [-]: specifies the start position in the output vector sent to the Sensor World
      | - Port dimensions [-]: specifies the width (number of scalars) of the output port
      | - Upload period [s]: specifies the upload period (in seconds) of the port.
      mask Display: port_label('input', 1, PortName)
  visu_TransWheelRR : Subsystem  mask(ToSensorWorld){PortName=visu_TransWheelRR_0, PortIndex=36, PortWidth=3, TimeStep=1/100}
      mask prompts: PortName "Port Name [-]"; PortIndex "Index [-]"; PortWidth "Port Dimensions [-]"; TimeStep "Upload Period [s]"
      mask help: Sends signal(s) from Simulink to the Sensor World
      mask Help:
      | Sends signal(s) from Simulink to the Sensor World.
      | 
      | - Port Name [-]: specifies the name of the output terminal of the Simulink block.
      | - Index [-]: specifies the start position in the output vector sent to the Sensor World
      | - Port dimensions [-]: specifies the width (number of scalars) of the output port
      | - Upload period [s]: specifies the upload period (in seconds) of the port.
      mask Display: port_label('input', 1, PortName)
  wires:
  conv_RotWheelRR/1(QuaternionVisu [rad]) -> visu_RotWheelRR/1(Y)
  conv_TransWheelRR/1(transVisu [m]) -> visu_TransWheelRR/1(Y)
  conv_RotWheelRL/1(QuaternionVisu [rad]) -> visu_RotWheelRL/1(Y)
  conv_TransWheelRL/1(transVisu [m]) -> visu_TransWheelRL/1(Y)
  conv_RotWheelFR/1(QuaternionVisu [rad]) -> visu_RotWheelFR/1(Y)
  conv_TransWheelFR/1(transVisu [m]) -> visu_TransWheelFR/1(Y)
  conv_RotWheelFL/1(QuaternionVisu [rad]) -> visu_RotWheelFL/1(Y)
  conv_TransWheelFL/1(transVisu [m]) -> visu_TransWheelFL/1(Y)
  Demux/8 -> Saturation5/1
  Demux/7 -> Saturation6/1
  Demux/6 -> Saturation3/1
  Demux/5 -> Saturation4/1
  Demux/4 -> Saturation1/1
  Demux/3 -> Saturation2/1
  Demux/2 -> Saturation8/1
  Demux/1 -> Saturation/1
  Saturation5/1 -> conv_RotWheelRR/1(BryantISO [deg])
  Saturation6/1 -> conv_TransWheelRR/1(transISO [m])
  Saturation3/1 -> conv_RotWheelRL/1(BryantISO [deg])
  Saturation4/1 -> conv_TransWheelRL/1(transISO [m])
  Saturation1/1 -> conv_RotWheelFR/1(BryantISO [deg])
  Saturation2/1 -> conv_TransWheelFR/1(transISO [m])
  Saturation8/1 -> conv_RotWheelFL/1(BryantISO [deg])
  Saturation/1 -> conv_TransWheelFL/1(transISO [m])
  Wheels/1 -> Demux/1  "wheels"
